simulink model "CSTR"  (R2025b)
settings: Solver=VariableStepAuto  StartTime=0.0  StopTime=10.0  RelTol=1e-3
undefined symbols (not defined in the file or in its folder): cfbar_sim, Tcbar_sim
settings Model: Creator=seby  LastModifiedBy=seby

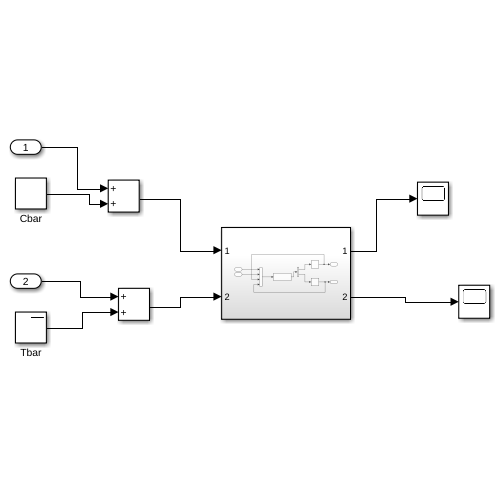
[thumbnail: Simulink's stored preview of the top-level diagram]
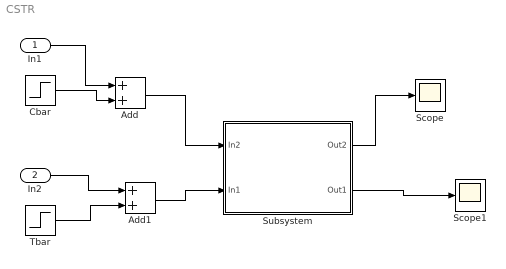
== system CSTR ==
  In1 : Inport
  In2 : Inport  Port=2
  Add : Sum
  Add1 : Sum
  Cbar : Step  After=cfbar_sim  SampleTime=0
  Scope : Scope
  Scope1 : Scope
  Subsystem : Subsystem
  Tbar : Step  After=Tcbar_sim  SampleTime=0
  wires:
  In1/1 -> Add/1
  Cbar/1 -> Add/2
  In2/1 -> Add1/1
  Tbar/1 -> Add1/2
  Add1/1 -> Subsystem/2(In1)
  Add/1 -> Subsystem/1(In2)
  Subsystem/2(Out1) -> Scope1/1
  Subsystem/1(Out2) -> Scope/1

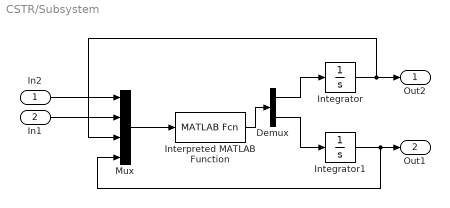
== system CSTR/Subsystem ==
  In2 : Inport
  In1 : Inport  Port=2
  Demux : Demux  Outputs=2
  Integrator : Integrator
  Integrator1 : Integrator
  Interpreted MATLAB Function : MATLABFcn
  Mux : Mux
  Out2 : Outport
  Out1 : Outport  Port=2
  wires:
  In1/1 -> Mux/2
  Mux/1 -> Interpreted MATLAB Function/1
  Interpreted MATLAB Function/1 -> Demux/1
  Demux/2 -> Integrator1/1
  Demux/1 -> Integrator/1
  Integrator1/1 -> Mux/4, Out1/1
  Integrator/1 -> Mux/3, Out2/1
  In2/1 -> Mux/1
